simulink model "PITCH_usporedba"  (R2020b)
settings: Solver=VariableStepAuto  StartTime=0.0  StopTime=10.0  RelTol=1e-3
undefined symbols (not defined in the file): k_p2, wn_p2, zeta_p2
settings Model: Creator=Ivan  LastModifiedBy=Ivan

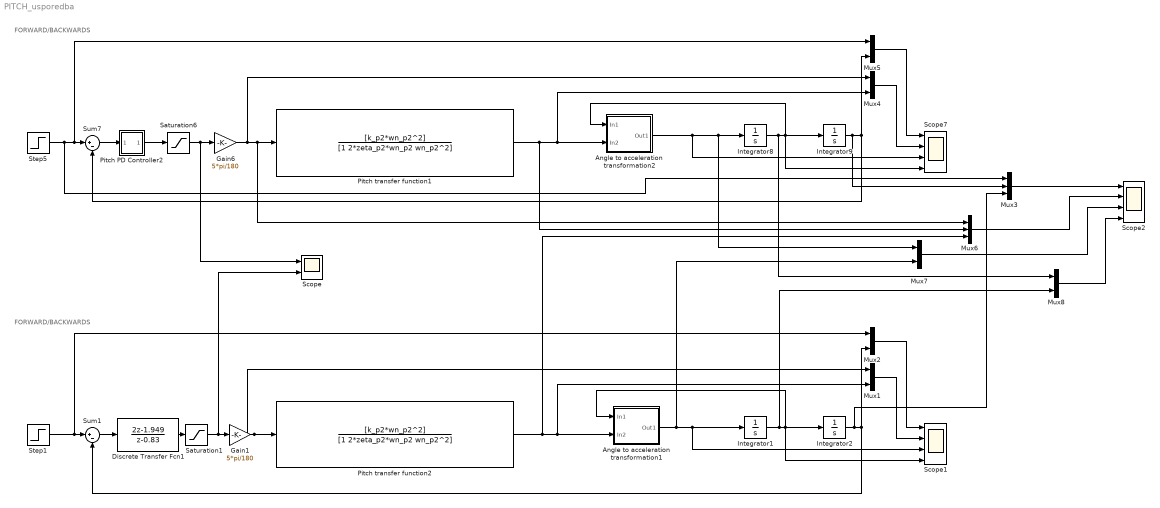
== system PITCH_usporedba ==
  note: FORWARD/BACKWARDS
  note: FORWARD/BACKWARDS
  Angle to acceleration transformation1 : Subsystem
  Angle to acceleration transformation2 : Subsystem
  Discrete Transfer Fcn1 : DiscreteTransferFcn  Numerator=[2 -1.949]  Denominator=[1 -0.83]  SampleTime=0.1
  Gain1 : Gain  Gain=5*pi/180
  Gain6 : Gain  Gain=5*pi/180
  Integrator{1..2,8..9} (4 alike) : Integrator
  Mux{1..2,4..5,7..8} (6 alike) : Mux  Inputs=2
  Mux3 : Mux  Inputs=3
  Mux6 : Mux  Inputs=3
  Pitch PD Controller2 : Subsystem
  Pitch transfer function1 : TransferFcn  Numerator=[k_p2*wn_p2^2]  Denominator=[1 2*zeta_p2*wn_p2 wn_p2^2]
  Pitch transfer function2 : TransferFcn  Numerator=[k_p2*wn_p2^2]  Denominator=[1 2*zeta_p2*wn_p2 wn_p2^2]
  Saturation1 : Saturate  UpperLimit=1  LowerLimit=-1
  Saturation6 : Saturate  UpperLimit=1  LowerLimit=-1
  Scope : Scope  NumInputPorts=2
  Scope1 : Scope  NumInputPorts=4
  Scope2 : Scope  NumInputPorts=4
  Scope7 : Scope  NumInputPorts=4
  Step1 : Step  Time=0  After=2  SampleTime=0
  Step5 : Step  Time=0  After=2  SampleTime=0
  Sum1 : Sum  Inputs=|+-
  Sum7 : Sum  Inputs=|+-
  wires:
  Saturation6/1 -> Scope/1, Gain6/1
  Pitch PD Controller2/1(" ") -> Saturation6/1
  Angle to acceleration transformation2/1(Out1) -> Scope7/3, Mux7/1, Integrator8/1
  Mux5/1 -> Scope7/1
  Mux4/1 -> Scope7/2
  Sum7/1 -> Pitch PD Controller2/1("  ")
  Step5/1 -> Mux3/1, Mux5/1, Sum7/1
  Integrator8/1 -> Mux8/1, Angle to acceleration transformation2/1(In1), Scope7/4, Integrator9/1
  Integrator9/1 -> Mux3/2, Mux5/2, Sum7/2
  Gain6/1 -> Mux4/1, Mux6/1, Pitch transfer function1/1
  Pitch transfer function1/1 -> Mux6/2, Mux4/2, Angle to acceleration transformation2/2(In2)
  Sum1/1 -> Discrete Transfer Fcn1/1
  Mux1/1 -> Scope1/2
  Step1/1 -> Mux2/1, Sum1/1
  Mux2/1 -> Scope1/1
  Discrete Transfer Fcn1/1 -> Saturation1/1
  Gain1/1 -> Mux1/1, Pitch transfer function2/1
  Integrator1/1 -> Mux8/2, Angle to acceleration transformation1/1(In1), Scope1/4, Integrator2/1
  Pitch transfer function2/1 -> Mux6/3, Mux1/2, Angle to acceleration transformation1/2(In2)
  Integrator2/1 -> Mux3/3, Mux2/2, Sum1/2
  Saturation1/1 -> Scope/2, Gain1/1
  Angle to acceleration transformation1/1(Out1) -> Mux7/2, Scope1/3, Integrator1/1
  Mux3/1 -> Scope2/1
  Mux6/1 -> Scope2/2
  Mux7/1 -> Scope2/3
  Mux8/1 -> Scope2/4

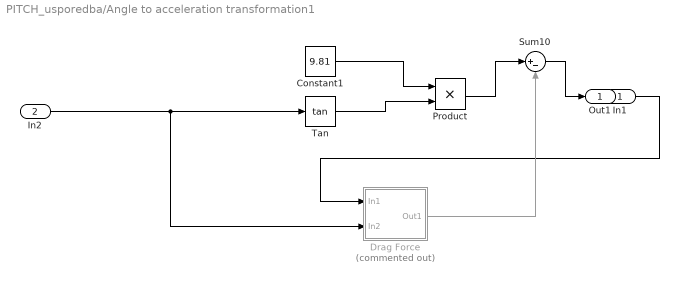
== system PITCH_usporedba/Angle to acceleration transformation1 ==
  In1 : Inport
  In2 : Inport  Port=2
  Constant1 : Constant  Value=9.81
  Drag Force : Subsystem  Commented=on
  Product : Product
  Sum10 : Sum  Inputs=|+-
  Tan : Trigonometry  Operator=tan
  Out1 : Outport
  wires:
  In2/1 -> Drag Force/2(In2), Tan/1
  Sum10/1 -> Out1/1
  Product/1 -> Sum10/1
  Tan/1 -> Product/2
  Constant1/1 -> Product/1
  In1/1 -> Drag Force/1(In1)
  Drag Force/1(Out1) -> Sum10/2

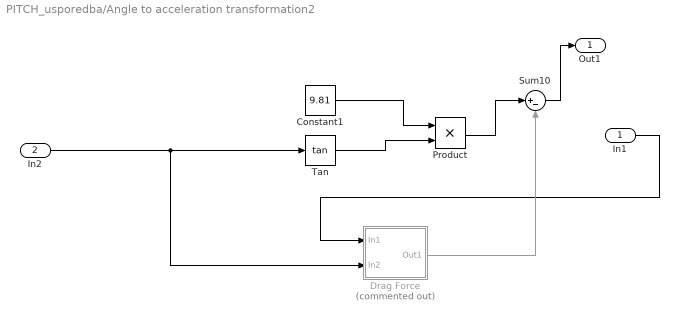
== system PITCH_usporedba/Angle to acceleration transformation2 ==
  In1 : Inport
  In2 : Inport  Port=2
  Constant1 : Constant  Value=9.81
  Drag Force : Subsystem  Commented=on
  Product : Product
  Sum10 : Sum  Inputs=|+-
  Tan : Trigonometry  Operator=tan
  Out1 : Outport
  wires:
  In2/1 -> Drag Force/2(In2), Tan/1
  Sum10/1 -> Out1/1
  Product/1 -> Sum10/1
  Tan/1 -> Product/2
  Constant1/1 -> Product/1
  In1/1 -> Drag Force/1(In1)
  Drag Force/1(Out1) -> Sum10/2

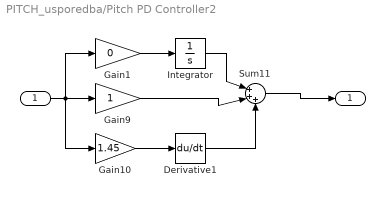
== system PITCH_usporedba/Pitch PD Controller2 ==
  "  " : Inport
  Derivative1 : Derivative
  Gain1 : Gain  Gain=0
  Gain10 : Gain  Gain=1.45
  Gain9 : Gain
  Integrator : Integrator
  Sum11 : Sum  Inputs=|+++
  " " : Outport
  wires:
  Sum11/1 -> " "/1
  Derivative1/1 -> Sum11/3
  "  "/1 -> Gain10/1, Gain1/1, Gain9/1
  Gain10/1 -> Derivative1/1
  Gain9/1 -> Sum11/2
  Integrator/1 -> Sum11/1
  Gain1/1 -> Integrator/1

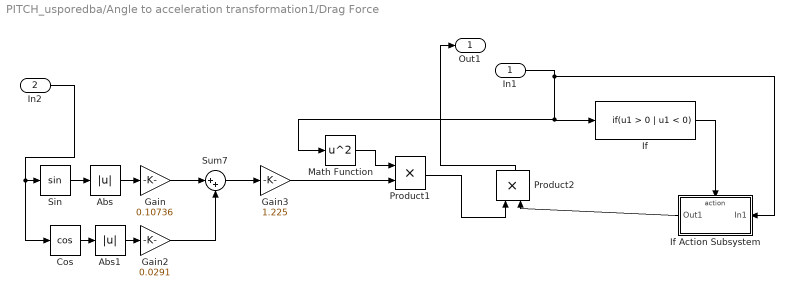
== system PITCH_usporedba/Angle to acceleration transformation1/Drag Force ==
  In1 : Inport
  In2 : Inport  Port=2
  Abs : Abs
  Abs1 : Abs
  Cos : Trigonometry  Operator=cos
  Gain : Gain  Gain=0.10736
  Gain2 : Gain  Gain=0.0291
  Gain3 : Gain  Gain=1.225
  If : If  IfExpression=u1 > 0 | u1 < 0  ShowElse=off
  If Action Subsystem : Subsystem  TreatAsAtomicUnit=on
  Math Function : Math  Operator=square  SaturateOnIntegerOverflow=on
  Product1 : Product
  Product2 : Product
  Sin : Trigonometry
  Sum7 : Sum  Inputs=|++
  Out1 : Outport
  wires:
  Cos/1 -> Abs1/1
  Abs/1 -> Gain/1
  Sum7/1 -> Gain3/1
  In1/1 -> If/1, Math Function/1, If Action Subsystem/1(In1)
  If Action Subsystem/1(Out1) -> Product2/2
  Sin/1 -> Abs/1
  In2/1 -> Sin/1, Cos/1
  Gain2/1 -> Sum7/2
  Math Function/1 -> Product1/1
  Abs1/1 -> Gain2/1
  Product1/1 -> Product2/1
  If/1 -> If Action Subsystem/Action
  Gain3/1 -> Product1/2
  Gain/1 -> Sum7/1
  Product2/1 -> Out1/1

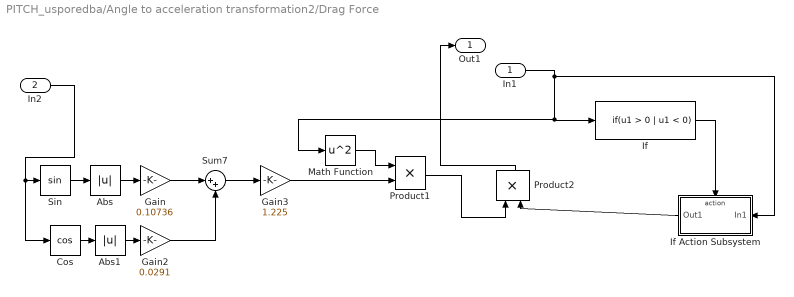
== system PITCH_usporedba/Angle to acceleration transformation2/Drag Force ==
  In1 : Inport
  In2 : Inport  Port=2
  Abs : Abs
  Abs1 : Abs
  Cos : Trigonometry  Operator=cos
  Gain : Gain  Gain=0.10736
  Gain2 : Gain  Gain=0.0291
  Gain3 : Gain  Gain=1.225
  If : If  IfExpression=u1 > 0 | u1 < 0  ShowElse=off
  If Action Subsystem : Subsystem  TreatAsAtomicUnit=on
  Math Function : Math  Operator=square  SaturateOnIntegerOverflow=on
  Product1 : Product
  Product2 : Product
  Sin : Trigonometry
  Sum7 : Sum  Inputs=|++
  Out1 : Outport
  wires:
  Cos/1 -> Abs1/1
  Abs/1 -> Gain/1
  Sum7/1 -> Gain3/1
  In1/1 -> If/1, Math Function/1, If Action Subsystem/1(In1)
  If Action Subsystem/1(Out1) -> Product2/2
  Sin/1 -> Abs/1
  In2/1 -> Sin/1, Cos/1
  Gain2/1 -> Sum7/2
  Math Function/1 -> Product1/1
  Abs1/1 -> Gain2/1
  Product1/1 -> Product2/1
  If/1 -> If Action Subsystem/Action
  Gain3/1 -> Product1/2
  Gain/1 -> Sum7/1
  Product2/1 -> Out1/1

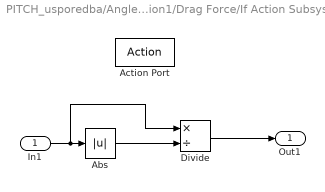
== system PITCH_usporedba/Angle to acceleration transformation1/Drag Force/If Action Subsystem ==
  In1 : Inport
  Action Port : ActionPort
  Abs : Abs
  Divide : Product  Inputs=*/
  Out1 : Outport
  wires:
  Divide/1 -> Out1/1
  In1/1 -> Abs/1, Divide/1
  Abs/1 -> Divide/2

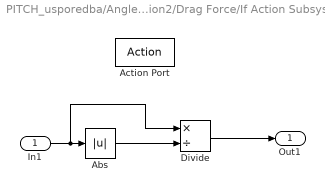
== system PITCH_usporedba/Angle to acceleration transformation2/Drag Force/If Action Subsystem ==
  In1 : Inport
  Action Port : ActionPort
  Abs : Abs
  Divide : Product  Inputs=*/
  Out1 : Outport
  wires:
  Divide/1 -> Out1/1
  In1/1 -> Abs/1, Divide/1
  Abs/1 -> Divide/2
